simulink model "mdl_with_State_Feedback_and_observer"  (R2025b)
settings: Solver=FixedStepAuto  StartTime=0.0  StopTime=Tsim  FixedStep=Ts  RelTol=1e-3
values from neighbouring files (symbols this model uses):
  IC = [0,deg2rad(1),0,0]    [Copy_of_main_final.m]
  input_select = [1,0]    [Copy_of_main_final.m]
  K = lqr(plant_ss.A, plant_ss.B, Q, R)    [Copy_of_main_final.m]    (also in test_anime.m = lqr(A, B, Q, Rw))
  k_scale = 1/dcg    [Copy_of_main_final.m]
  L = params.L    [test_anime.m]
  plant_ss = plant_ss_q1    [Copy_of_main_final.m]    (also in syst_repr_generator.m = ss(A,B,C,D))
  plant_ss_diag = diagonalize(plant_ss)    [Copy_of_main_final.m]    (also in diagonalize.m = ss(A_d, B_d, C_d, 0))
  q2_f = deg2rad(10)    [Copy_of_main_final.m]
undefined symbols (not defined in the file or in its folder): params
libraries: SignalEditorBlockLib x1
settings Model: Creator=dsagn  LastModifiedBy=dsagn
settings SolverCC: AlgebraicLoopSolver=TrustRegion
settings DataIOCC: ReturnWorkspaceOutputs=off
settings DebuggingCC: UnconnectedInputMsg=warning  UnconnectedOutputMsg=warning  UnconnectedLineMsg=warning  ArithmeticOperatorsInVariantConditions=warning
settings ModelReferenceCC: EnableRefExpFcnMdlSchedulingChecks=on
settings SFSimCC: CustomCodeUndefinedFunction=UseInterfaceOnly
settings RTWCC: GPUComputeCapability=3.5

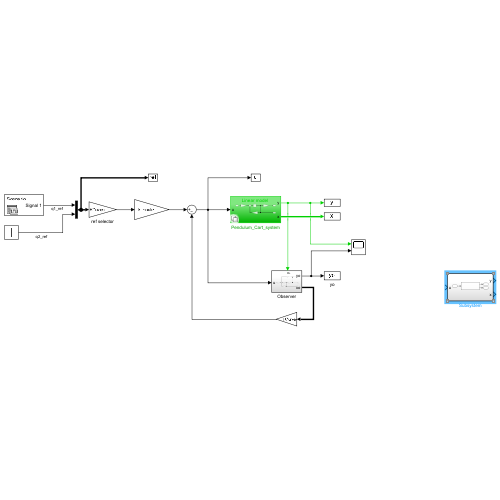
[thumbnail: Simulink's stored preview of the top-level diagram]
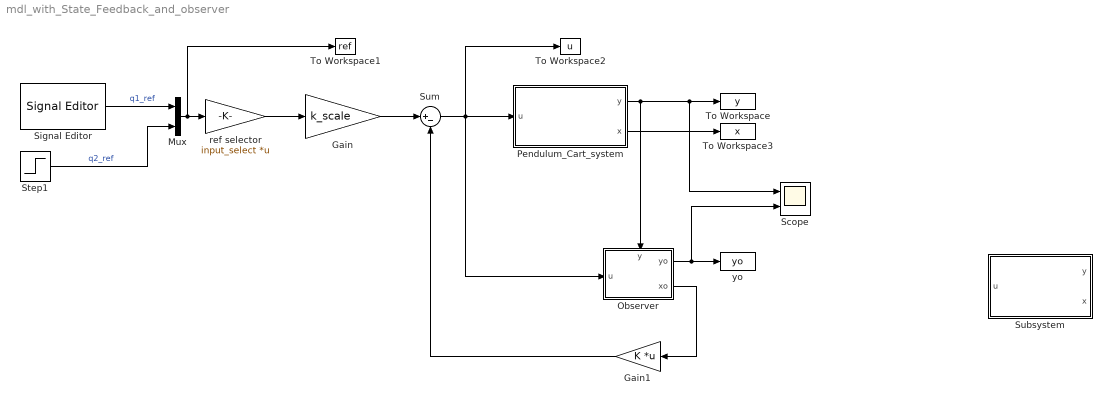
== system mdl_with_State_Feedback_and_observer ==
  Gain : Gain  Gain=k_scale
  Gain1 : Gain  Gain=K  Multiplication=Matrix(K*u) (u vector)
  Mux : Mux  Inputs=2
  Observer : Subsystem  VariantControl=model==1
      settings: PortSchema="{\"entries\":[{\"content\":{\"sides\":[{\"content\":{\"connectorIds\":[\"In1\"]},\"type\":\"ConnectorPlacement.EquallySpacedRectSide\",\"uuid\":\"6f29056e-8395-4acf-a958-2cc2da83c6bb\"},{\"content\":{\"connectorIds\":[\"Out1\",\"Out2\"],\"side\":\"RIGHT\"},\"type\":\"ConnectorPlacement.EquallySpacedRectSide\",\"uuid\":\"2e81148d-cd4e-4b0e-acc4-d8b2ace90135\"},{\"content\":{\"connectorIds\":[\"In2\"],\"side\":\"TOP\"},\"type\":\"ConnectorPlacement.EquallySpacedRectSide\",\"uuid\":\"710f508c-edb8-4863-9098-12d33f6e7baf\"},{\"content\":{\"side\":\"BOTTOM\"},\"type\":\"ConnectorPlacement.EquallySpacedRectSide\",\"uuid\":\"bc3670e7-573f-4e2e-9d5c-9aa118a3e582\"}]},\"type\":\"ConnectorPlacement.EquallySpacedConnector\",\"uuid\":\"432a14f0-84c3-4e6e-8c18-6f5dc974cf86\"}],\"packageUris\":[\"http://schema.mathworks.com/mf0/Connector/R2020b\"],\"version\":\"1.0\"}"
  Pendulum_Cart_system : Subsystem  Variant=on
  Scope : Scope  NumInputPorts=2
      settings: ActiveDisplayYMinimum=-1  ActiveDisplayYMaximum=1
  Signal Editor : SignalEditorBlockLib/Signal Editor  FileName=q1_scenario1.mat  ActiveScenario=Scenario  ActiveSignal=Signal 1  IsBus=off  OutputBusObjectStr=Bus: BusObject  SampleTime=0  ZeroCross=off  OutputAfterFinalValue=Setting to zero  Unit=inherit  PreserveSignalName=on  ApplySigPropsToAllScenarios=on  ApplySigPropsToAllSignals=off  SignalPropertySource=Dialog parameters
  Step1 : Step  After=q2_f  SampleTime=0
  Subsystem : Subsystem
  Sum : Sum  Inputs=|+-
  To Workspace : ToWorkspace  VariableName=y  SaveFormat=Timeseries  SampleTime=-1
  To Workspace1 : ToWorkspace  VariableName=ref  SaveFormat=Timeseries  SampleTime=-1
  To Workspace2 : ToWorkspace  VariableName=u  SaveFormat=Timeseries  SampleTime=-1
  To Workspace3 : ToWorkspace  VariableName=x  SaveFormat=Timeseries  SampleTime=-1
  ref selector : Gain  Gain=input_select  Multiplication=Matrix(K*u) (u vector)
  yo : ToWorkspace  VariableName=yo  SaveFormat=Timeseries  SampleTime=-1
  wires:
  ref selector/1 -> Gain/1
  Pendulum_Cart_system/2(x) -> To Workspace3/1
  Pendulum_Cart_system/1(y) -> Scope/1, To Workspace/1, Observer/2(y)
  Step1/1 -> Mux/2  "q2_ref"
  Mux/1 -> To Workspace1/1, ref selector/1
  Signal Editor/1 -> Mux/1  "q1_ref"
  Gain1/1 -> Sum/2
  Gain/1 -> Sum/1
  Sum/1 -> To Workspace2/1, Observer/1(u), Pendulum_Cart_system/1(u)
  Observer/2(xo) -> Gain1/1
  Observer/1(yo) -> Scope/2, yo/1

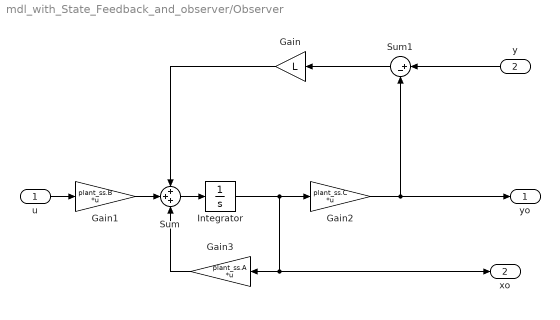
== system mdl_with_State_Feedback_and_observer/Observer ==
  u : Inport
  y : Inport  Port=2
  Gain : Gain  Gain=L
  Gain1 : Gain  Gain=plant_ss.B  Multiplication=Matrix(K*u) (u vector)
  Gain2 : Gain  Gain=plant_ss.C  Multiplication=Matrix(K*u) (u vector)
  Gain3 : Gain  Gain=plant_ss.A  Multiplication=Matrix(K*u) (u vector)
  Integrator : Integrator  InitialCondition=IC
  Sum : Sum  Inputs=+++
  Sum1 : Sum  Inputs=|+-
  yo : Outport
  xo : Outport  Port=2
  wires:
  u/1 -> Gain1/1
  Gain1/1 -> Sum/2
  Sum/1 -> Integrator/1
  Gain3/1 -> Sum/3
  Integrator/1 -> Gain2/1, Gain3/1, xo/1
  Gain2/1 -> yo/1, Sum1/2
  Sum1/1 -> Gain/1
  y/1 -> Sum1/1
  Gain/1 -> Sum/1

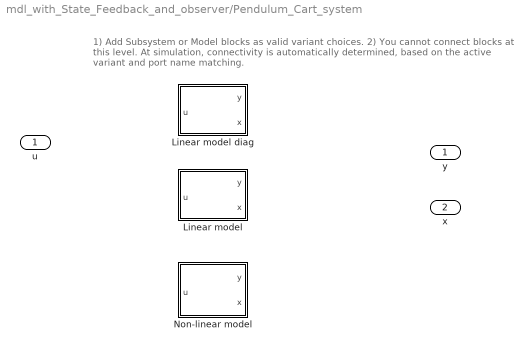
== system mdl_with_State_Feedback_and_observer/Pendulum_Cart_system ==
  note: 1) Add Subsystem or Model blocks as valid variant choices.
      | 2) You cannot connect blocks at this level. At simulation, connectivity is automatically
      | determined, based on the active variant and port name matching.
  u : Inport
  "Linear model " : Subsystem  VariantControl=model==1
  Linear model diag : Subsystem  VariantControl=model==2
  Non-linear model : Subsystem  VariantControl=model==3
  y : Outport
  x : Outport  Port=2

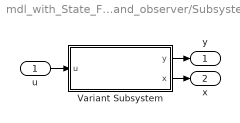
== system mdl_with_State_Feedback_and_observer/Subsystem ==
  u : Inport
  Variant Subsystem : Subsystem  Variant=on
  y : Outport
  x : Outport  Port=2
  wires:
  Variant Subsystem/2(x) -> x/1
  u/1 -> Variant Subsystem/1(u)
  Variant Subsystem/1(y) -> y/1

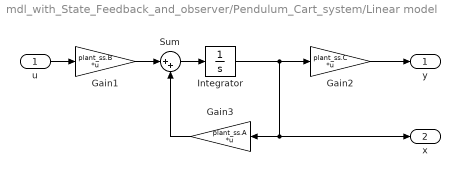
== system mdl_with_State_Feedback_and_observer/Pendulum_Cart_system/Linear model  ==
  u : Inport
  Gain1 : Gain  Gain=plant_ss.B  Multiplication=Matrix(K*u) (u vector)
  Gain2 : Gain  Gain=plant_ss.C  Multiplication=Matrix(K*u) (u vector)
  Gain3 : Gain  Gain=plant_ss.A  Multiplication=Matrix(K*u) (u vector)
  Integrator : Integrator  InitialCondition=IC
  Sum : Sum  Inputs=|++
  y : Outport
  x : Outport  Port=2
  wires:
  u/1 -> Gain1/1
  Gain1/1 -> Sum/1
  Sum/1 -> Integrator/1
  Gain3/1 -> Sum/2
  Integrator/1 -> Gain2/1, Gain3/1, x/1
  Gain2/1 -> y/1

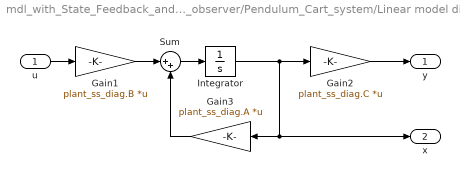
== system mdl_with_State_Feedback_and_observer/Pendulum_Cart_system/Linear model diag ==
  u : Inport
  Gain1 : Gain  Gain=plant_ss_diag.B  Multiplication=Matrix(K*u) (u vector)
  Gain2 : Gain  Gain=plant_ss_diag.C  Multiplication=Matrix(K*u) (u vector)
  Gain3 : Gain  Gain=plant_ss_diag.A  Multiplication=Matrix(K*u) (u vector)
  Integrator : Integrator  InitialCondition=IC
  Sum : Sum  Inputs=|++
  y : Outport
  x : Outport  Port=2
  wires:
  Gain2/1 -> y/1
  Integrator/1 -> x/1, Gain3/1, Gain2/1
  Gain3/1 -> Sum/2
  Sum/1 -> Integrator/1
  Gain1/1 -> Sum/1
  u/1 -> Gain1/1

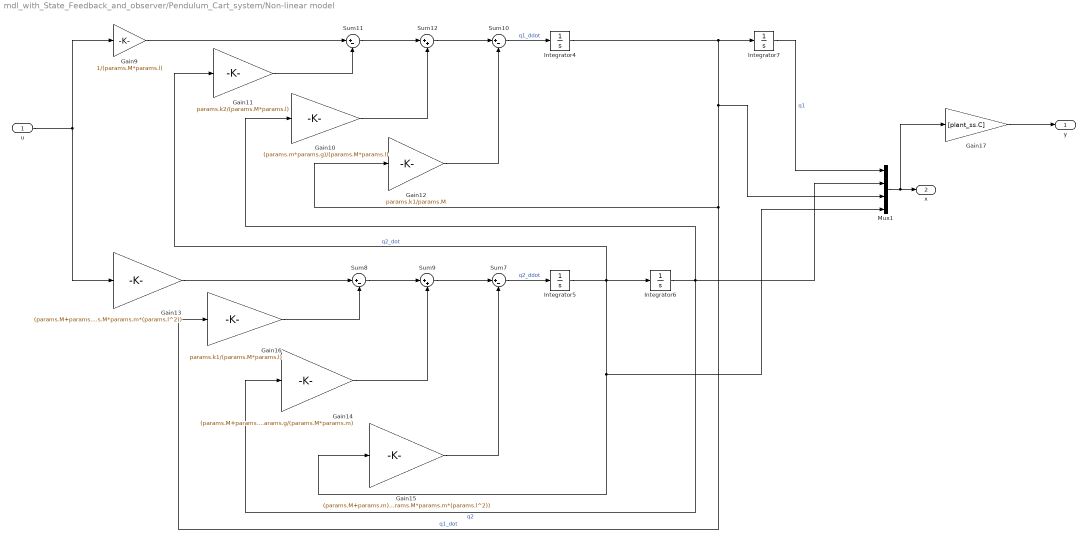
== system mdl_with_State_Feedback_and_observer/Pendulum_Cart_system/Non-linear model ==
  u : Inport
  Gain10 : Gain  Gain=(params.m*params.g)/(params.M*params.l)
  Gain11 : Gain  Gain=params.k2/(params.M*params.l)
  Gain12 : Gain  Gain=params.k1/params.M
  Gain13 : Gain  Gain=(params.M+params.m)/(params.M*params.m*(params.l^2))
  Gain14 : Gain  Gain=(params.M+params.m)*params.g/(params.M*params.m)
  Gain15 : Gain  Gain=(params.M+params.m)*params.k2/(params.M*params.m*(params.l^2))
  Gain16 : Gain  Gain=params.k1/(params.M*params.l)
  Gain17 : Gain  Gain=[plant_ss.C]
  Gain9 : Gain  Gain=1/(params.M*params.l)
  Integrator4 : Integrator
  Integrator5 : Integrator
  Integrator6 : Integrator  InitialCondition=IC(2)
  Integrator7 : Integrator
  Mux1 : Mux
  Sum{7..8,10..11} (4 alike) : Sum  Inputs=|+-
  Sum12 : Sum  Inputs=|++
  Sum9 : Sum  Inputs=|++
  y : Outport  VectorParamsAs1DForOutWhenUnconnected=off
  x : Outport  Port=2
  wires:
  Gain16/1 -> Sum8/2
  Integrator6/1 -> Mux1/2, Gain14/1, Gain10/1  "q2"
  Sum8/1 -> Sum9/1
  Integrator7/1 -> Mux1/1  "q1"
  Gain12/1 -> Sum10/2
  Sum10/1 -> Integrator4/1  "q1_ddot"
  u/1 -> Gain13/1, Gain9/1
  Gain14/1 -> Sum9/2
  Integrator5/1 -> Mux1/4, Gain15/1, Gain11/1, Integrator6/1  "q2_dot"
  Mux1/1 -> Gain17/1, x/1
  Sum9/1 -> Sum7/1
  Sum7/1 -> Integrator5/1  "q2_ddot"
  Sum11/1 -> Sum12/1
  Sum12/1 -> Sum10/1
  Gain10/1 -> Sum12/2
  Gain17/1 -> y/1
  Gain11/1 -> Sum11/2
  Gain9/1 -> Sum11/1
  Gain15/1 -> Sum7/2
  Integrator4/1 -> Integrator7/1, Mux1/3, Gain16/1, Gain12/1  "q1_dot"
  Gain13/1 -> Sum8/1

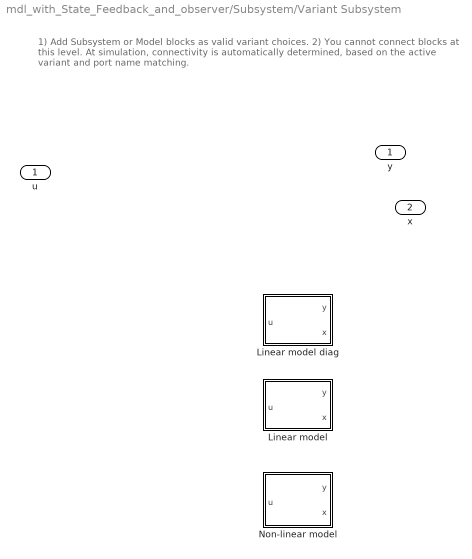
== system mdl_with_State_Feedback_and_observer/Subsystem/Variant Subsystem ==
  note: 1) Add Subsystem or Model blocks as valid variant choices.
      | 2) You cannot connect blocks at this level. At simulation, connectivity is automatically
      | determined, based on the active variant and port name matching.
  u : Inport
  "Linear model " : Subsystem  VariantControl=model==1
  Linear model diag : Subsystem  VariantControl=model==2
  Non-linear model : Subsystem  VariantControl=model==3
  y : Outport
  x : Outport  Port=2

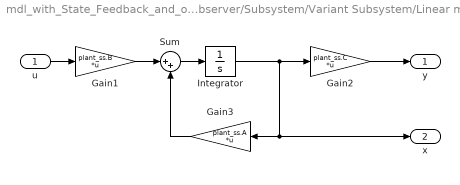
== system mdl_with_State_Feedback_and_observer/Subsystem/Variant Subsystem/Linear model  ==
  u : Inport
  Gain1 : Gain  Gain=plant_ss.B  Multiplication=Matrix(K*u) (u vector)
  Gain2 : Gain  Gain=plant_ss.C  Multiplication=Matrix(K*u) (u vector)
  Gain3 : Gain  Gain=plant_ss.A  Multiplication=Matrix(K*u) (u vector)
  Integrator : Integrator  InitialCondition=IC
  Sum : Sum  Inputs=|++
  y : Outport
  x : Outport  Port=2
  wires:
  u/1 -> Gain1/1
  Gain1/1 -> Sum/1
  Sum/1 -> Integrator/1
  Gain3/1 -> Sum/2
  Integrator/1 -> Gain2/1, Gain3/1, x/1
  Gain2/1 -> y/1

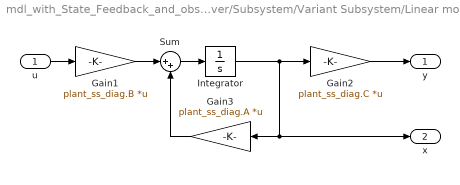
== system mdl_with_State_Feedback_and_observer/Subsystem/Variant Subsystem/Linear model diag ==
  u : Inport
  Gain1 : Gain  Gain=plant_ss_diag.B  Multiplication=Matrix(K*u) (u vector)
  Gain2 : Gain  Gain=plant_ss_diag.C  Multiplication=Matrix(K*u) (u vector)
  Gain3 : Gain  Gain=plant_ss_diag.A  Multiplication=Matrix(K*u) (u vector)
  Integrator : Integrator  InitialCondition=IC
  Sum : Sum  Inputs=|++
  y : Outport
  x : Outport  Port=2
  wires:
  Gain2/1 -> y/1
  Integrator/1 -> x/1, Gain3/1, Gain2/1
  Gain3/1 -> Sum/2
  Sum/1 -> Integrator/1
  Gain1/1 -> Sum/1
  u/1 -> Gain1/1

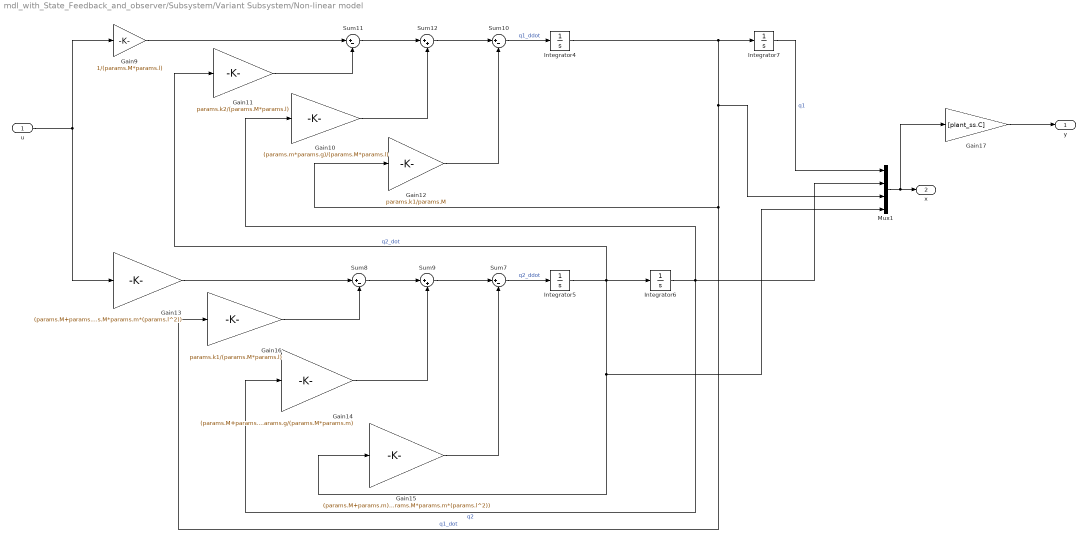
== system mdl_with_State_Feedback_and_observer/Subsystem/Variant Subsystem/Non-linear model ==
  u : Inport
  Gain10 : Gain  Gain=(params.m*params.g)/(params.M*params.l)
  Gain11 : Gain  Gain=params.k2/(params.M*params.l)
  Gain12 : Gain  Gain=params.k1/params.M
  Gain13 : Gain  Gain=(params.M+params.m)/(params.M*params.m*(params.l^2))
  Gain14 : Gain  Gain=(params.M+params.m)*params.g/(params.M*params.m)
  Gain15 : Gain  Gain=(params.M+params.m)*params.k2/(params.M*params.m*(params.l^2))
  Gain16 : Gain  Gain=params.k1/(params.M*params.l)
  Gain17 : Gain  Gain=[plant_ss.C]
  Gain9 : Gain  Gain=1/(params.M*params.l)
  Integrator4 : Integrator
  Integrator5 : Integrator
  Integrator6 : Integrator  InitialCondition=IC(2)
  Integrator7 : Integrator
  Mux1 : Mux
  Sum{7..8,10..11} (4 alike) : Sum  Inputs=|+-
  Sum12 : Sum  Inputs=|++
  Sum9 : Sum  Inputs=|++
  y : Outport  VectorParamsAs1DForOutWhenUnconnected=off
  x : Outport  Port=2
  wires:
  Gain16/1 -> Sum8/2
  Integrator6/1 -> Mux1/2, Gain14/1, Gain10/1  "q2"
  Sum8/1 -> Sum9/1
  Integrator7/1 -> Mux1/1  "q1"
  Gain12/1 -> Sum10/2
  Sum10/1 -> Integrator4/1  "q1_ddot"
  u/1 -> Gain13/1, Gain9/1
  Gain14/1 -> Sum9/2
  Integrator5/1 -> Mux1/4, Gain15/1, Gain11/1, Integrator6/1  "q2_dot"
  Mux1/1 -> Gain17/1, x/1
  Sum9/1 -> Sum7/1
  Sum7/1 -> Integrator5/1  "q2_ddot"
  Sum11/1 -> Sum12/1
  Sum12/1 -> Sum10/1
  Gain10/1 -> Sum12/2
  Gain17/1 -> y/1
  Gain11/1 -> Sum11/2
  Gain9/1 -> Sum11/1
  Gain15/1 -> Sum7/2
  Integrator4/1 -> Integrator7/1, Mux1/3, Gain16/1, Gain12/1  "q1_dot"
  Gain13/1 -> Sum8/1
